simulink model "Mu_synthesis_quarter_car"  (R2025b)
settings: Solver=VariableStepAuto  StartTime=0.0  StopTime=10  RelTol=1e-3
values from neighbouring files (symbols this model uses):
  omega_n1 = 80    [A_quarter_car_parameters.m]    (also in A_uncertain_Plant.m = parameters.omega_n1; Incert_plant.m; LQG.m; LQG_pt2.m)
  tau_1 = 0.005    [A_quarter_car_parameters.m]    (also in LQG.m; LQG_pt2.m; LQG_pt2.mat; Lin_model.m)
  tau_2 = 0.010    (= 0.01)    [A_quarter_car_parameters.m]    (also in LQG.m; LQG_pt2.m; LQG_pt2.mat; Lin_model.m)
  tau_a = 0.025    [A_quarter_car_parameters.m]    (also in A_uncertain_Plant.m = parameters.tau_a; Incert_plant.m; LQG.m; LQG_pt2.m)
  x0_delta_s = 0    [A_quarter_car_parameters.m]    (also in quarter_car_parameters.m)
  x0_delta_t = 0    [A_quarter_car_parameters.m]    (also in quarter_car_parameters.m)
  x0_zs_dot = 0    [A_quarter_car_parameters.m]    (also in quarter_car_parameters.m)
  x0_zu_dot = 0    [A_quarter_car_parameters.m]    (also in quarter_car_parameters.m)
  zeta_1 = 0.7    [A_quarter_car_parameters.m]    (also in A_uncertain_Plant.m = parameters.zeta_1; Incert_plant.m; LQG.m; LQG_pt2.m)
libraries: simulink x4, cstblocks x2
settings Model: Creator=ettor  LastModifiedBy=ettor

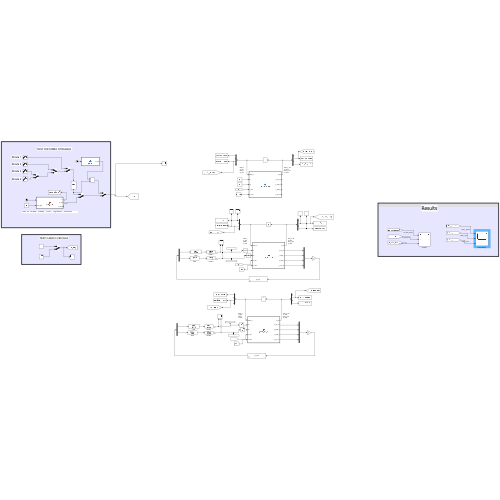
[thumbnail: Simulink's stored preview of the top-level diagram]
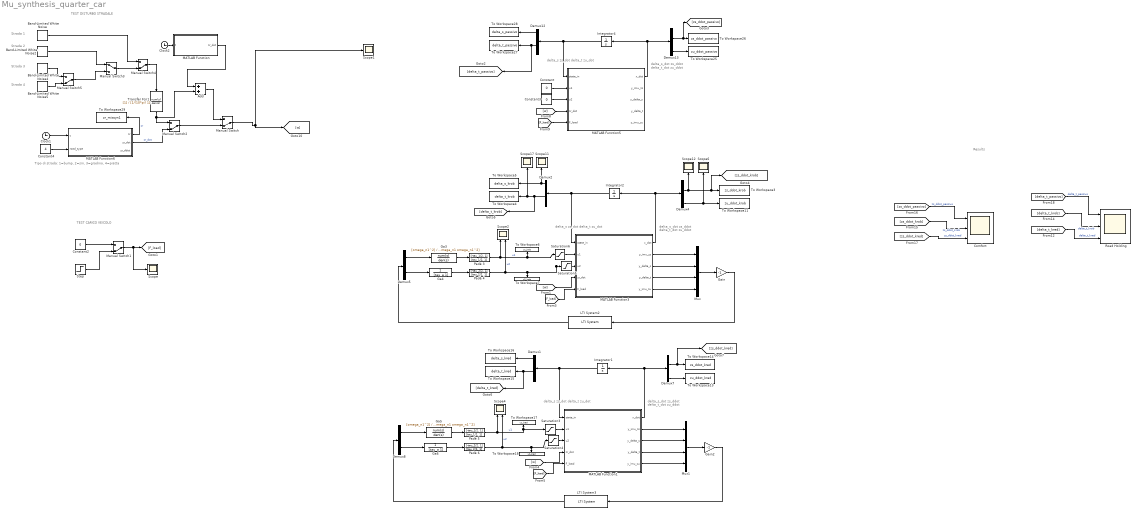
== system Mu_synthesis_quarter_car ==
  note: Strada 2
  note: Tipo di strada: 1=bump, 2=sin, 3=gradino, 4=piatta
  note: TEST DISTURBO STRADALE
  note: Strada 3
  note: delta_s_dot
      | zs_ddot
      | delta_t_dot
      | zu_ddot
  note: Results
  note: TEST CARICO VEICOLO
  note: delta_s
      | zs_dot
      | delta_t
      | zu_dot
  note: delta_s_dot
      | zs_ddot
      | delta_t_dot
      | zu_ddot
  note: Strada 4
  note: delta_s_dot
      | zs_ddot
      | delta_t_dot
      | zu_ddot
  note: delta_s
      | zs_dot
      | delta_t
      | zu_dot
  note: Strada 1
  note: delta_s
      | zs_dot
      | delta_t
      | zu_dot
  Add : Sum
  Band-Limited White Noise : simulink/Sources/Band-Limited White Noise  Cov=[5e-3*0.01]  Ts=0.01  seed=[23341]
  Band-Limited White Noise2 : simulink/Sources/Band-Limited White Noise  Cov=[6e-2*0.01]  Ts=0.01  seed=[23341]
  Band-Limited White Noise4 : simulink/Sources/Band-Limited White Noise  Cov=[0.15*0.01]  Ts=0.01  seed=[23341]
  Band-Limited White Noise5 : simulink/Sources/Band-Limited White Noise  Cov=[0.30*0.01]  Ts=0.01  seed=[23341]
  Clock1 : Clock
  Clock2 : Clock
  "Comfort " : Scope  NumInputPorts=3
      settings: ActiveDisplayYMinimum=-6.7481571046929236  ActiveDisplayYMaximum=6.8388810633239183  YLabel=[m/s^2]  DataLoggingVariableName=ScopeData20
  Constant : Constant  Value=0
  Constant2 : Constant  Value=0
  Constant3 : Constant  Value=0
  Constant4 : Constant  Value=4
  Demux{1..2,4,7,12..13} (6 alike) : Demux
  Demux5 : Demux  Outputs=2
  Demux8 : Demux  Outputs=2
  Ga3 : TransferFcn  Numerator=[omega_n1^2]  Denominator=[1 2*zeta_1*omega_n1 omega_n1^2]
  Ga4 : TransferFcn  Denominator=[tau_a 1]
  Ga5 : TransferFcn  Numerator=[omega_n1^2]  Denominator=[1 2*zeta_1*omega_n1 omega_n1^2]
  Ga6 : TransferFcn  Denominator=[tau_a 1]
  Gain : Gain  Gain=-1
  Gain2 : Gain  Gain=-1
  Integrator1 : Integrator  InitialCondition=[x0_delta_s; x0_zs_dot; x0_delta_t; x0_zu_dot]
  Integrator2 : Integrator  InitialCondition=[x0_delta_s; x0_zs_dot; x0_delta_t; x0_zu_dot]
  Integrator4 : Integrator  InitialCondition=[x0_delta_s; x0_zs_dot; x0_delta_t; x0_zu_dot]
  LTI System2 : cstblocks/LTI System  sys=K_rob  IC=[]  PadeOrder=0
  LTI System3 : cstblocks/LTI System  sys=K_red  IC=[]  PadeOrder=0
  MATLAB Function : MATLAB Function  TreatAsAtomicUnit=on
  MATLAB Function1 : MATLAB Function  TreatAsAtomicUnit=on
  MATLAB Function3 : MATLAB Function  TreatAsAtomicUnit=on
  MATLAB Function5 : MATLAB Function  TreatAsAtomicUnit=on
  MATLAB Function6 : MATLAB Function  TreatAsAtomicUnit=on
  Manual Switch{,1..2,4..5} (5 alike) : ManualSwitch  CurrentSetting=0
  Manual Switch3 : ManualSwitch
  Mux : Mux
  Mux1 : Mux
  Padè 3 : TransferFcn  Numerator=[-tau_1/2, 1]  Denominator=[tau_1/2, 1]
  Padè 4 : TransferFcn  Numerator=[-tau_2/2, 1]  Denominator=[tau_2/2, 1]
  Padè 5 : TransferFcn  Numerator=[-tau_1/2, 1]  Denominator=[tau_1/2, 1]
  Padè 6 : TransferFcn  Numerator=[-tau_2/2, 1]  Denominator=[tau_2/2, 1]
  "Road Holding " : Scope  NumInputPorts=3
      settings: ActiveDisplayYMinimum=-0.035666702308631157  ActiveDisplayYMaximum=0.0364748029964308  YLabel=[m]  DataLoggingVariableName=ScopeData21
  Saturation{3..6} (4 alike) : Saturate  UpperLimit=+3000  LowerLimit=-3000
  Scope{,1,6,11..12,17} (6 alike) : Scope
      Scope settings: ActiveDisplayYMinimum=-1  ActiveDisplayYMaximum=1
      Scope1 settings: ActiveDisplayYMinimum=-1  ActiveDisplayYMaximum=1
      Scope11 settings: ActiveDisplayYMinimum=-0.097286960700178962  ActiveDisplayYMaximum=0.041921688545787351  DataLoggingVariableName=ScopeData11
      Scope12 settings: ActiveDisplayYMinimum=-8.1092984788503877  ActiveDisplayYMaximum=7.1261344945484675  DataLoggingVariableName=ScopeData12
      Scope17 settings: ActiveDisplayYMinimum=-0.032931521848176631  ActiveDisplayYMaximum=0.034866157724541193  DataLoggingVariableName=ScopeData17
      Scope6 settings: ActiveDisplayYMinimum=-8.1092984788503877  ActiveDisplayYMaximum=7.1261344945484675  DataLoggingVariableName=ScopeData6
  Scope2 : Scope  NumInputPorts=2
      settings: ActiveDisplayYMinimum=-5655.3016129165408  ActiveDisplayYMaximum=4157.4442581158046  DataLoggingVariableName=ScopeData2
  Scope4 : Scope  NumInputPorts=2
      settings: ActiveDisplayYMinimum=-2385.206123263566  ActiveDisplayYMaximum=606.27783975154966  DataLoggingVariableName=ScopeData4
  Step : Step  Time=2  After=500  SampleTime=0
  To Workspace11 : ToWorkspace  VariableName=zu_ddot_krob  SaveFormat=Timeseries  SampleTime=-1
  To Workspace13 : ToWorkspace  VariableName=zu_ddot_kred  SaveFormat=Timeseries  SampleTime=-1
  To Workspace14 : ToWorkspace  VariableName=zs_ddot_kred  SaveFormat=Timeseries  SampleTime=-1
  To Workspace15 : ToWorkspace  VariableName=delta_t_kred  SaveFormat=Timeseries  SampleTime=-1
  To Workspace16 : ToWorkspace  VariableName=delta_s_kred  SaveFormat=Timeseries  SampleTime=-1
  To Workspace17 : ToWorkspace  VariableName=u1_kred  SaveFormat=Timeseries  SampleTime=-1
  To Workspace18 : ToWorkspace  VariableName=u2_kred  SaveFormat=Timeseries  SampleTime=-1
  To Workspace25 : ToWorkspace  VariableName=zu_ddot_passivo  SaveFormat=Timeseries  SampleTime=-1
  To Workspace26 : ToWorkspace  VariableName=zs_ddot_passivo  SaveFormat=Timeseries  SampleTime=-1
  To Workspace27 : ToWorkspace  VariableName=delta_t_passivo  SaveFormat=Timeseries  SampleTime=-1
  To Workspace28 : ToWorkspace  VariableName=delta_s_passivo  SaveFormat=Timeseries  SampleTime=-1
  To Workspace29 : ToWorkspace  VariableName=zr_mixsyn1  SaveFormat=Timeseries  SampleTime=-1
  To Workspace3 : ToWorkspace  VariableName=zs_ddot_krob  SaveFormat=Timeseries  SampleTime=-1
  To Workspace4 : ToWorkspace  VariableName=delta_t_krob  SaveFormat=Timeseries  SampleTime=-1
  To Workspace5 : ToWorkspace  VariableName=delta_s_krob  SaveFormat=Timeseries  SampleTime=-1
  To Workspace6 : ToWorkspace  VariableName=u1_krob  SaveFormat=Timeseries  SampleTime=-1
  To Workspace7 : ToWorkspace  VariableName=u2_krob  SaveFormat=Timeseries  SampleTime=-1
  Transfer Fcn1 : TransferFcn  Denominator=[1/(10*pi) 1]
  wires:
  [delta_t_kred] -> "Road Holding "/3  "delta_t_kred"
  Manual Switch5/1 -> Manual Switch3/2
  Transfer Fcn1/1 -> Add/2, Manual Switch2/1
  Band-Limited White Noise4/1 -> Manual Switch5/1
  Clock1/1 -> MATLAB Function6/1(t)
  Band-Limited White Noise5/1 -> Manual Switch5/2
  Constant4/1 -> MATLAB Function6/2(road_type)
  Band-Limited White Noise2/1 -> Manual Switch3/1
  Manual Switch4/1 -> Transfer Fcn1/1
  MATLAB Function6/2(zr_dot) -> Manual Switch2/2  "zr_dot"
  [delta_t_passivo] -> "Road Holding "/1  "delta_t_passivo"
  [delta_t_krob] -> "Road Holding "/2  "delta_t_krob"
  [zs_ddot_kred] -> "Comfort "/3  "zs_ddot_kred"
  Demux8/2 -> Ga6/1
  Demux5/2 -> Ga4/1
  Ga3/1 -> Padè 3/1
  Demux1/1 -> To Workspace16/1
  [zs_ddot_krob] -> "Comfort "/2  "zs_ddot_krob"
  Integrator2/1 -> MATLAB Function3/1(state_in), Demux2/1
  MATLAB Function3/3(y_delta_s) -> Mux/2
  LTI System2/1 -> Demux5/1
  MATLAB Function1/4(y_delta_t) -> Mux1/3
  Demux2/1 -> To Workspace5/1, Scope11/1
  [zs_ddot_passivo] -> "Comfort "/1  "zs_ddot_passivo"
  MATLAB Function1/5(y_imu_zu) -> Mux1/4
  [w] -> MATLAB Function5/4(zr_dot)
  MATLAB Function6/1(zr) -> To Workspace29/1  "zr"
  Padè 5/1 -> Saturation3/1, To Workspace17/1, Scope4/1  "u1"
  Integrator1/1 -> MATLAB Function1/1(state_in), Demux1/1
  Ga5/1 -> Padè 5/1
  [F_load] -> MATLAB Function1/5(F_load)
  Saturation3/1 -> MATLAB Function1/2(u1)
  Demux2/3 -> [delta_t_krob], To Workspace4/1, Scope17/1
  Ga4/1 -> Padè 4/1
  MATLAB Function3/2(y_imu_zs) -> Mux/1
  Demux4/2 -> Scope12/1, [zs_ddot_krob], To Workspace3/1
  Manual Switch3/1 -> Manual Switch4/2
  [w] -> MATLAB Function3/4(zr_dot)
  MATLAB Function3/1(x_dot) -> Demux4/1, Integrator2/1
  Constant2/1 -> Manual Switch1/1
  Padè 6/1 -> Saturation4/1, To Workspace18/1, Scope4/2  "u2"
  Demux4/4 -> Scope6/1, To Workspace11/1
  Constant/1 -> MATLAB Function5/2(u1)
  MATLAB Function1/2(y_imu_zs) -> Mux1/1
  Padè 3/1 -> To Workspace6/1, Saturation6/1, Scope2/1  "u1"
  [F_load] -> MATLAB Function5/5(F_load)
  Demux7/4 -> To Workspace13/1
  Band-Limited White Noise/1 -> Manual Switch4/1
  Demux12/1 -> To Workspace28/1
  Step/1 -> Manual Switch1/2
  Demux5/1 -> Ga3/1
  MATLAB Function1/3(y_delta_s) -> Mux1/2
  Gain2/1 -> LTI System3/1
  Demux7/2 -> [zs_ddot_kred], To Workspace14/1
  Mux/1 -> Gain/1
  Demux13/2 -> [zs_ddot_passivo], To Workspace26/1
  MATLAB Function3/4(y_delta_t) -> Mux/3
  Demux8/1 -> Ga5/1
  Demux1/3 -> [delta_t_kred], To Workspace15/1
  Ga6/1 -> Padè 6/1
  Padè 4/1 -> MATLAB Function3/3(u2), Saturation5/1, To Workspace7/1, Scope2/2  "u2"
  MATLAB Function3/5(y_imu_zu) -> Mux/4
  Saturation4/1 -> MATLAB Function1/3(u2)
  Mux1/1 -> Gain2/1
  [F_load] -> MATLAB Function3/5(F_load)
  Demux13/4 -> To Workspace25/1
  Saturation6/1 -> MATLAB Function3/2(u1)
  Demux12/3 -> To Workspace27/1, [delta_t_passivo]
  Gain/1 -> LTI System2/1
  Integrator4/1 -> MATLAB Function5/1(state_in), Demux12/1
  Manual Switch1/1 -> Scope/1, [F_load]
  Constant3/1 -> MATLAB Function5/3(u2)
  MATLAB Function5/1(x_dot) -> Demux13/1, Integrator4/1
  [w] -> MATLAB Function1/4(zr_dot)
  LTI System3/1 -> Demux8/1
  MATLAB Function1/1(x_dot) -> Demux7/1, Integrator1/1
  MATLAB Function/1(zr_dot) -> Add/1
  Clock2/1 -> MATLAB Function/1(t)
  Add/1 -> Manual Switch/1
  Manual Switch/1 -> Scope1/1, [w]
  Manual Switch2/1 -> Manual Switch/2

== matlab function Mu_synthesis_quarter_car/MATLAB Function1 ==
  data: state_in input; x_dot output; u1 input; u2 input; zr_dot input; F_load input; parameters parameter; y_imu_zs output; y_delta_s output; y_delta_t output; y_imu_zu output
function [x_dot, y_imu_zs, y_delta_s, y_delta_t, y_imu_zu] = quarter_car_NL(state_in, u1, u2, zr_dot, F_load ,parameters)

    delta_s = state_in(1);
    zs_dot = state_in(2);
    delta_t = state_in(3);
    zu_dot = state_in(4);
    
    m_s = parameters.m_s;
    m_u = parameters.m_u;
    ks0 = parameters.ks0;
    alpha = parameters.alpha;
    bs = parameters.bs;
    kt = parameters.kt;
    bt = parameters.bt;
    
    delta_s_dot = zs_dot - zu_dot;
    delta_t_dot = zu_dot - zr_dot;
    
    Fs = ks0 * delta_s + alpha * delta_s^3 + bs * delta_s_dot;
    Ft = kt * delta_t + bt * delta_t_dot;
    
    
    zs_ddot = (-Fs + u1-F_load) / m_s;
    zu_ddot = (Fs - Ft - u1 + u2) / m_u;
    
    x_dot = [delta_s_dot; zs_ddot; delta_t_dot; zu_ddot];
    
    y_imu_zs = zs_ddot;  
    y_imu_zu = zu_ddot; 
    y_delta_s = delta_s; 
    y_delta_t = delta_t; 

end

== matlab function Mu_synthesis_quarter_car/MATLAB Function ==
  data: t input; zr_dot output; params parameter
function zr_dot  = bump(t, params)


    A = params.A;   % altezza [m]
    L = params.L;   % lunghezza [m]
    v = params.v;   % velocità veicolo [m/s]
    t0 = 5; % istante di inizio ostacolo [s]
    T = L / v;      % durata temporale bump
            
    % Il dosso inizia a t0 e finisce a t0 + T
    if t >= t0 && t <= (t0 + T)
        t_rel = t - t0; % Tempo relativo (parte da 0 quando inizia il dosso)
        phi   = 2*pi*v*t_rel / L;
        zr    = (A/2) * (1 - cos(phi));
        zr_dot   = (A*pi*v/L) * sin(phi);
        zr_ddot  = (A*2*pi^2*v^2/L^2) * cos(phi);
    else
        zr = 0;  zr_dot = 0;  zr_ddot = 0;
    end
end

== matlab function Mu_synthesis_quarter_car/MATLAB Function3 ==
  data: state_in input; x_dot output; u1 input; u2 input; zr_dot input; F_load input; parameters parameter; y_imu_zs output; y_delta_s output; y_delta_t output; y_imu_zu output
function [x_dot, y_imu_zs, y_delta_s, y_delta_t, y_imu_zu] = quarter_car_NL(state_in, u1, u2, zr_dot, F_load ,parameters)

    delta_s = state_in(1);
    zs_dot = state_in(2);
    delta_t = state_in(3);
    zu_dot = state_in(4);
    
    m_s = parameters.m_s;
    m_u = parameters.m_u;
    ks0 = parameters.ks0;
    alpha = parameters.alpha;
    bs = parameters.bs;
    kt = parameters.kt;
    bt = parameters.bt;
    
    delta_s_dot = zs_dot - zu_dot;
    delta_t_dot = zu_dot - zr_dot;
    
    Fs = ks0 * delta_s + alpha * delta_s^3 + bs * delta_s_dot;
    Ft = kt * delta_t + bt * delta_t_dot;
    
    
    zs_ddot = (-Fs + u1-F_load) / m_s;
    zu_ddot = (Fs - Ft - u1 + u2) / m_u;
    
    x_dot = [delta_s_dot; zs_ddot; delta_t_dot; zu_ddot];
    
    y_imu_zs = zs_ddot;  
    y_imu_zu = zu_ddot; 
    y_delta_s = delta_s; 
    y_delta_t = delta_t; 

end

== matlab function Mu_synthesis_quarter_car/MATLAB Function5 ==
  data: state_in input; x_dot output; u1 input; u2 input; zr_dot input; F_load input; parameters parameter; y_imu_zs output; y_delta_s output; y_delta_t output; y_imu_zu output
function [x_dot, y_imu_zs, y_delta_s, y_delta_t, y_imu_zu] = quarter_car_NL(state_in, u1, u2, zr_dot, F_load ,parameters)

    delta_s = state_in(1);
    zs_dot = state_in(2);
    delta_t = state_in(3);
    zu_dot = state_in(4);
    
    m_s = parameters.m_s;
    m_u = parameters.m_u;
    ks0 = parameters.ks0;
    alpha = parameters.alpha;
    bs = parameters.bs;
    kt = parameters.kt;
    bt = parameters.bt;
    
    delta_s_dot = zs_dot - zu_dot;
    delta_t_dot = zu_dot - zr_dot;
    
    Fs = ks0 * delta_s + alpha * delta_s^3 + bs * delta_s_dot;
    Ft = kt * delta_t + bt * delta_t_dot;
    
    
    zs_ddot = (-Fs + u1-F_load) / m_s;
    zu_ddot = (Fs - Ft - u1 + u2) / m_u;
    
    x_dot = [delta_s_dot; zs_ddot; delta_t_dot; zu_ddot];
    
    y_imu_zs = zs_ddot;  
    y_imu_zu = zu_ddot; 
    y_delta_s = delta_s; 
    y_delta_t = delta_t; 

end

== matlab function Mu_synthesis_quarter_car/MATLAB Function6 ==
  data: t input; zr output; zr_dot output; zr_ddot output; params parameter; road_type input
function [zr, zr_dot, zr_ddot] = road_profile(t, params, road_type)
%   road_type = 1 bump | 2 sinusoide | 3 gradino | 4 piatta

    switch road_type
        case 1  % ---- BUMP ----

            A = params.A;   % altezza [m]
            L = params.L;   % lunghezza [m]
            v = params.v;   % velocità veicolo [m/s]
            t0 = params.t0; % istante di inizio ostacolo [s]
            T = L / v;      % durata temporale bump
            
            % Il dosso inizia a t0 e finisce a t0 + T
            if t >= t0 && t <= (t0 + T)
                t_rel = t - t0; % Tempo relativo (parte da 0 quando inizia il dosso)
                phi   = 2*pi*v*t_rel / L;
                zr    = (A/2) * (1 - cos(phi));
                zr_dot   = (A*pi*v/L) * sin(phi);
                zr_ddot  = (A*2*pi^2*v^2/L^2) * cos(phi);
            else
                zr = 0;  zr_dot = 0;  zr_ddot = 0;
            end
            
        case 2  % ---- SINUSOIDE ----
            A = params.A;   % ampiezza [m]
            f = params.f;   % frequenza [Hz]
            t0 = params.t0; % istante di inizio ostacolo [s]
            
            % La strada vibra solo dopo t0
            if t >= t0
                t_rel = t - t0; % Tempo relativo
                w = 2*pi*f;
                zr   =  A * sin(w*t_rel);
                zr_dot  =  A * w * cos(w*t_rel);
                zr_ddot = -A * w^2 * sin(w*t_rel);
            else
                zr = 0;  zr_dot = 0;  zr_ddot = 0;
            end
            
        case 3  % ---- GRADINO SMUSSATO ----
            A  = params.A;    % altezza [m]
            t0 = params.t0;   % istante del gradino [s]
            tau = params.tau/1000; % tempo di salita [s]
            
            arg  = (t - t0) / tau;
            zr   = (A/2) * (1 + tanh(arg));
            zr_dot  = (A/(2*tau)) * (sech(arg))^2;
            zr_ddot = -(A/tau^2) * (sech(arg))^2 * tanh(arg);
            
        case 4  % ---- STRADA PIATTA ----
            zr = 0;  zr_dot = 0;  zr_ddot = 0;
            
        otherwise 
            zr = 0;  zr_dot = 0;  zr_ddot = 0;
    end
end
